simulink model "extractLocal_sim"  (R2024b)
settings: Solver=VariableStepAuto  StartTime=0.0  StopTime=10.0  RelTol=1e-3
InitFcn:
  | extractLocalMapSetup
undefined symbols (not defined in the file): tuneableTEBParams, worldGridLoc, worldMat, worldRes
libraries: simulink x1, roshelperlib x1
settings Model: Creator=cstabile  LastModifiedBy=jbrault
settings SolverCC: DateTimeAtSimulationTimeZero=[]

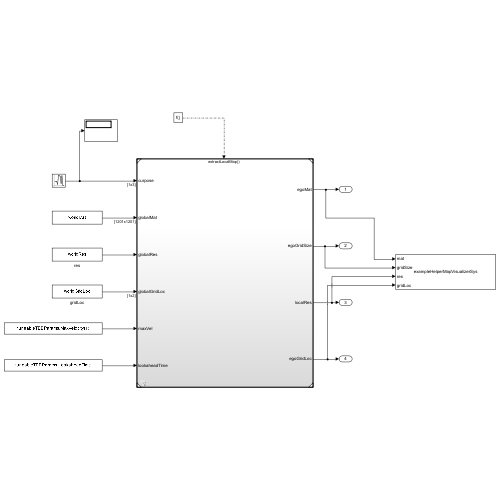
[thumbnail: Simulink's stored preview of the top-level diagram]
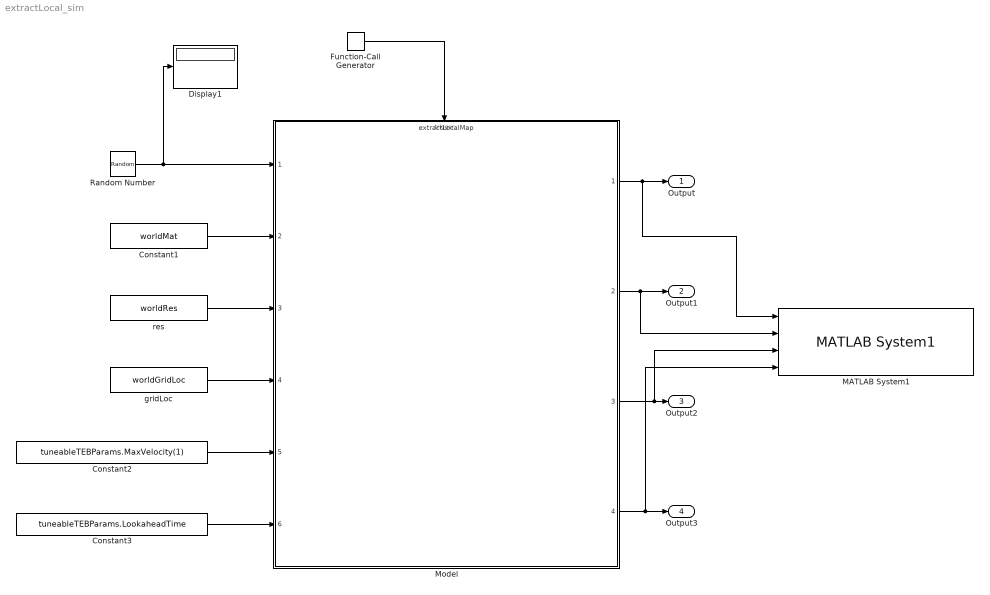
== system extractLocal_sim ==
  Constant1 : Constant  Value=worldMat
  Constant2 : Constant  Value=tuneableTEBParams.MaxVelocity(1)
  Constant3 : Constant  Value=tuneableTEBParams.LookaheadTime
  Display1 : Display
  Function-Call Generator : simulink/Ports & Subsystems/Function-Call Generator  sample_time=1  numberOfIterations=1  DisallowWideOutput=off
  MATLAB System1 : roshelperlib/MATLAB System1  MapType=SDF  IsEgo=off  DisplayVisual=on  SimulateUsing=Interpreted execution
  Model : ModelReference  ModelNameDialog=extractLocalMap.slx  SimulationMode=Normal  ModelReferenceVersion=2.0  TriggerPortName=function  TriggerPortTriggerType=function-call  TriggerPortStatesWhenEnabling=held
  Random Number : RandomNumber  Mean=[500 500 0]  Variance=[100 100 0]
  gridLoc : Constant  Value=worldGridLoc  VectorParams1D=off
  res : Constant  Value=worldRes
  Output : Outport
  Output1 : Outport  Port=2
  Output2 : Outport  Port=3
  Output3 : Outport  Port=4
  wires:
  Random Number/1 -> Display1/1, Model/1
  Constant1/1 -> Model/2
  res/1 -> Model/3
  gridLoc/1 -> Model/4
  Model/1 -> MATLAB System1/1, Output/1
  Constant2/1 -> Model/5
  Model/3 -> MATLAB System1/3, Output2/1
  Constant3/1 -> Model/6
  Model/2 -> MATLAB System1/2, Output1/1
  Model/4 -> MATLAB System1/4, Output3/1
  Function-Call Generator/1 -> Model/Trigger
